simulink model "PI_Controller"  (R2020b)
settings: Solver=ode45  StartTime=0.0  StopTime=120  RelTol=1e-3
values from neighbouring files (symbols this model uses):
  Ki = 20    [Variables.m]
  Kp = 10    [Variables.m]
  Ts = 0.1    [Variables.m]
settings Model: Creator=samar  LastModifiedBy=samar
settings DataIOCC: SaveOutput=off  SaveTime=off

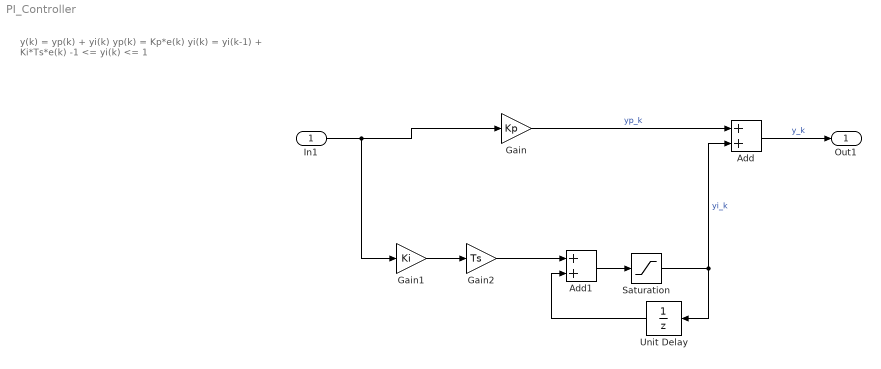
== system PI_Controller ==
  note: y(k) = yp(k) + yi(k)
      |
      | yp(k) = Kp*e(k)
      |
      | yi(k) = yi(k-1) + Ki*Ts*e(k)
      |
      | -1 <= yi(k) <= 1
  In1 : Inport  OutDataTypeStr=double  PortDimensions=1  SampleTime=0
  Add : Sum
  Add1 : Sum
  Gain : Gain  Gain=Kp
  Gain1 : Gain  Gain=Ki
  Gain2 : Gain  Gain=Ts
  Saturation : Saturate  UpperLimit=1  LowerLimit=-1
  Unit Delay : UnitDelay  SampleTime=-1  HasFrameUpgradeWarning=on
  Out1 : Outport  OutDataTypeStr=double  PortDimensions=1  SampleTime=0
  wires:
  Saturation/1 -> Add/2, Unit Delay/1  "yi_k"
  Gain/1 -> Add/1  "yp_k"
  Gain1/1 -> Gain2/1
  Add/1 -> Out1/1  "y_k"
  Unit Delay/1 -> Add1/2
  In1/1 -> Gain1/1, Gain/1
  Gain2/1 -> Add1/1
  Add1/1 -> Saturation/1
